simulink model "MATMPC_SIMULINK_R2017b"  (R2021b)
settings: Solver=FixedStepAuto  StartTime=0.0  StopTime=4.0  RelTol=1e-3
InitFcn:
  | Initialization_Simulink
values from neighbouring files (symbols this model uses):
  Ts = settings.Ts_st    [Initialization_Simulink.m]    (also in Simulation.m)
  x0 = input.x0    [Initialization_Simulink.m]
undefined symbols (not defined in the file or in its folder): opt, settings
settings Model: Creator=chen  LastModifiedBy=enric
settings SolverCC: AlgebraicLoopSolver=TrustRegion
settings DataIOCC: ReturnWorkspaceOutputs=off
settings DebuggingCC: SFMachineParentedDataDiag=warning  ArithmeticOperatorsInVariantConditions=warning
settings SFSimCC: SimUseLocalCustomCode=off  CustomCodeUndefinedFunction=UseInterfaceOnly
settings RTWCC: RTWUseLocalCustomCode=off  CheckMdlBeforeBuild=Error

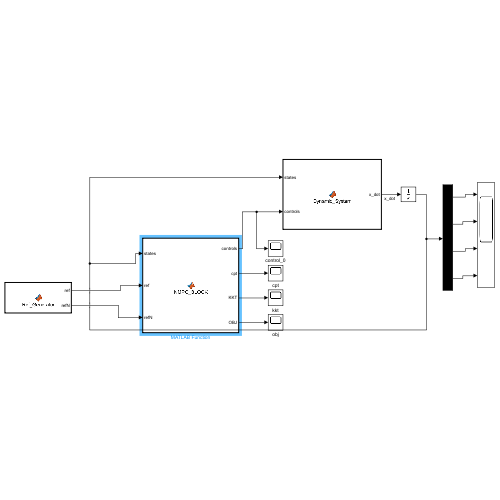
[thumbnail: Simulink's stored preview of the top-level diagram]
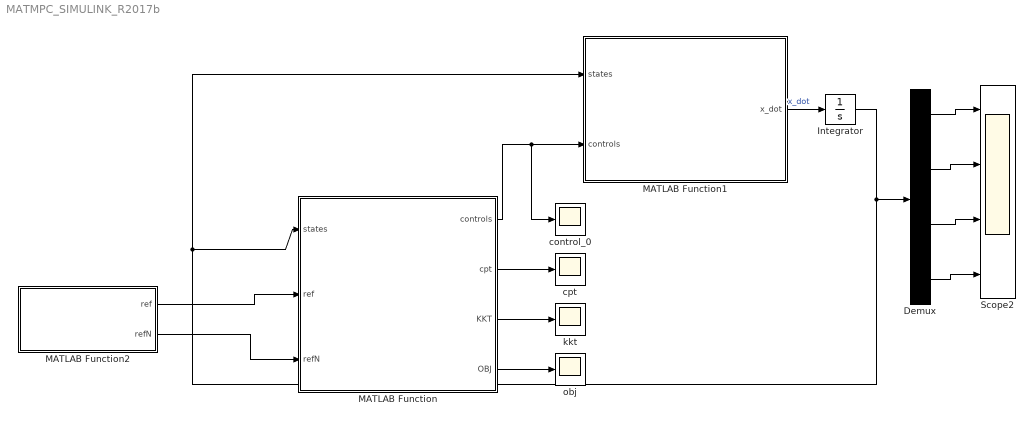
== system MATMPC_SIMULINK_R2017b ==
  Demux : Demux
  Integrator : Integrator  InitialCondition=x0
  MATLAB Function : MATLAB Function  TreatAsAtomicUnit=on  SystemSampleTime=Ts
  MATLAB Function1 : MATLAB Function  TreatAsAtomicUnit=on
  MATLAB Function2 : MATLAB Function  TreatAsAtomicUnit=on
  Scope2 : Scope  NumInputPorts=4
  control_0 : Scope
  cpt : Scope
  kkt : Scope
  obj : Scope
  wires:
  MATLAB Function/1(controls) -> control_0/1, MATLAB Function1/2(controls)
  MATLAB Function1/1(x_dot) -> Integrator/1  "x_dot"
  Integrator/1 -> Demux/1, MATLAB Function/1(states), MATLAB Function1/1(states)
  Demux/1 -> Scope2/1
  Demux/2 -> Scope2/2
  Demux/3 -> Scope2/3
  Demux/4 -> Scope2/4
  MATLAB Function/2(cpt) -> cpt/1
  MATLAB Function/4(OBJ) -> obj/1
  MATLAB Function/3(KKT) -> kkt/1
  MATLAB Function2/1(ref) -> MATLAB Function/2(ref)
  MATLAB Function2/2(refN) -> MATLAB Function/3(refN)

== matlab function MATMPC_SIMULINK_R2017b/MATLAB Function1 ==
  data: states input size=nx; x_dot output size=nx; controls input size=nu
function x_dot  = Dynamic_System(states,controls)

M = 1; 
m = 0.1;
l = 0.8; 
g = 9.81;

p=states(1);
theta=states(2);
v=states(3);
omega=states(4);  
u=controls(1);

a=-m*l*sin(theta)*omega^2+m*g*cos(theta)*sin(theta)+u;
b=-m*l*cos(theta)*sin(theta)*omega^2+u*cos(theta)+(M+m)*g*sin(theta);
c=M+m-m*(cos(theta))^2;

x_dot = [v;omega;a/c;b/(l*c)];

return

== matlab function MATMPC_SIMULINK_R2017b/MATLAB Function ==
  settings: updateMethod=DISCRETE
  data: states input size=nx; controls output size=nu; cpt output size=1; settings parameter; opt parameter; ref input size=[ny N]; KKT output; OBJ output; refN input size=nyN
function [controls, cpt, KKT, OBJ] = NMPC_BLOCK(states, settings, opt, ref, refN)

%% everything should has a fixed size
coder.extrinsic('mpc_nmpcsolver');  
coder.extrinsic('InitData'); 
coder.extrinsic('InitData_ngrid'); 
coder.extrinsic('InitMemory');  
coder.extrinsic('evalin');
coder.extrinsic('assignin');

%%

%#codegen

persistent x u lambda mu mu_x mu_u;
persistent input mem;

if isempty(input)  
nx = settings.nx;        % No. of states
    nz = settings.nz;        % No. of algebraic states
    nu = settings.nu;        % No. of controls
    ny = settings.ny;        % No. of outputs (references)    
    nyN= settings.nyN;       % No. of outputs at terminal stage 
    np = settings.np;        % No. of parameters (on-line data)
    nc = settings.nc;        % No. of constraints
    ncN = settings.ncN;      % No. of constraints at terminal stage
    nbu = settings.nbu;      % No. of control bounds
    nbx = settings.nbx;      % No. of state bounds
    nbu_idx = settings.nbu_idx; % Index of control bounds
    nbx_idx = settings.nbx_idx; % Index of state bounds
    N = settings.N;
    N2 = settings.N2;
    r = settings.r;
        
    input.x0=zeros(nx,1);
    input.z0=zeros(nz,1);
    
    x=repmat(input.x0,1,N+1);
    input.x=x;
    if nz>0
        input.z0=zeros(nz,1);
        input.z=zeros(nz,N);
    else
        input.z0=0;
        input.z=0;
    end
    u=zeros(nu,N);
    input.u=u;
    
    lambda = zeros(nx,N+1);
    input.lambda= lambda;
    
    if N*nc+ncN > 0
        mu = zeros(N*nc+ncN,1);
    else
        mu = 0;
    end
    input.mu= mu;
    
    mu_u = zeros(N*nu,1);
    input.mu_u= mu_u;
    
    if N*nbx > 0
        mu_x = zeros(N*nbx,1);
    else
        mu_x = 0;
    end
    input.mu_x = mu_x;
    
    input.W=repmat(zeros(ny,1),1,N);
    input.WN=zeros(nyN,1);
    input.od = repmat(zeros(np,1),1,N+1);
    
    if nc>0
        input.lb = [repmat(zeros(nc,1),N,1);zeros(ncN,1)];
        input.ub = [repmat(zeros(nc,1),N,1);zeros(ncN,1)];
    else
        input.lb=0;
        input.ub=0;
    end

    if nbx>0
        input.lbx = repmat(zeros(nbx,1),1,N+1);
        input.ubx = repmat(zeros(nbx,1),1,N+1);
    else
        input.lbx=0;
        input.ubx=0;
    end

    lbu = -inf(nu,1);
    ubu = inf(nu,1);
    lb_u = zeros(nbu,1);
    ub_u = zeros(nbu,1);
    for i=1:nbu
        lbu(nbu_idx(i)) = lb_u(i);
        ubu(nbu_idx(i)) = ub_u(i);
    end
    input.lbu = repmat(lbu,1,N);
    input.ubu = repmat(ubu,1,N);
      
    input.y = zeros(ny,N);
    input.yN = zeros(nyN,1);

    input.info.cpuTime=0;
    input.info.OptCrit=0;
    input.info.objValue=0;

%     if opt.nonuniform_grid
%         [input, ~] = InitData_ngrid(settings);
%         N = r;
%         settings.N = N;
%     else
        [input, ~] = InitData(settings);
%     end
%     
    mem = InitMemory(settings, opt, input);

%     input = evalin('base','input');
%     mem = evalin('base','mem');
        
else

    input.x=x; 
    input.u=u;
    input.lambda=lambda;   
    input.mu=mu;
    input.mu_x=mu_x;
    input.mu_u=mu_u;
    
end

%%

input.x0 = states;
[input,mem] = mpc_nmpcsolver(input, settings, mem, opt);
% cpt,KKT,OBJ
cpt=input.info.cpuTime;
KKT=input.info.OptCrit;
OBJ=input.info.objValue;
controls = input.u(1,1);

%% shifting
switch opt.shifting
    case 'yes'
        x=[input.x(:,2:end),input.x(:,end)];  
        u=[input.u(:,2:end),input.u(:,end)]; 
        lambda=[input.lambda(:,2:end),input.lambda(:,end)];
        if (settings.N*settings.nc+settings.ncN) >0
            mu(1:end-settings.ncN+1)=input.mu(settings.nc+1:settings.N*settings.nc+settings.ncN,1);
            mu(settings.N*settings.nc+1:end)=input.mu(settings.N*settings.nc+settings.ncN-settings.nc+1:settings.N*settings.nc+settings.ncN,1);
        else
            mu=0;
        end
        mu_x=[input.mu_x(2:end,1);input.mu_x(end,1)];
        mu_u=[input.mu_u(2:end,1);input.mu_u(end,1)];
   case 'no'
        x=input.x;
        u=input.u;
        lambda=input.lambda;
        mu=input.mu;
        mu_x=input.mu_x;
        mu_u=input.mu_u;
end

return

== matlab function MATMPC_SIMULINK_R2017b/MATLAB Function2 ==
  data: ref output; settings parameter; refN output
function [ref,refN] = Ref_Generator(  settings)

ref=zeros(settings.ny,settings.N);
refN=zeros(settings.nyN,1);
